simulink model "Sixteen_June_Sensors"  (R2022a)
settings: Solver=FixedStepAuto  StartTime=0.0  StopTime=80  RelTol=1e-3
settings Model: ExtModeTrigDuration=80  Creator=DevGunu  LastModifiedBy=DevGunu
settings OptimizationCC: EnhancedBackFolding=on  PassReuseOutputArgsAs=Individual arguments  ZeroExternalMemoryAtStartup=off  ZeroInternalMemoryAtStartup=off  MaxStackSize=64  OptimizeBlockOrder=speed  DifferentSizesBufferReuse=on  OptimizationCustomize=off  EfficientTunableParamExpr=on
settings DebuggingCC: ParameterTunabilityLossMsg=error
settings HardwareCC: ProdBitPerPointer=32  ProdBitPerSizeT=32  ProdBitPerPtrDiffT=32  ProdLargestAtomicInteger=Long  ProdWordSize=32  ProdHWDeviceType=ARM Compatible->ARM 9  UseEmbeddedCoderFeatures=off
settings SFSimCC: MATLABDynamicMemAlloc=off
settings RTWCC: SystemTargetFile=ert.tlc  HardwareBoard=PARROT Mambo  TemplateMakefile=ert_default_tmf  Toolchain=Sourcery G++ Lite GNU Toolchain for Drones
settings CodeAppCC: ForceParamTrailComments=on  IgnoreCustomStorageClasses=off  OperatorAnnotations=on  SimulinkDataObjDesc=on  SFDataObjDesc=on  InsertBlockDesc=on
settings ERTTargetCC: SupportNonInlinedSFcns=on

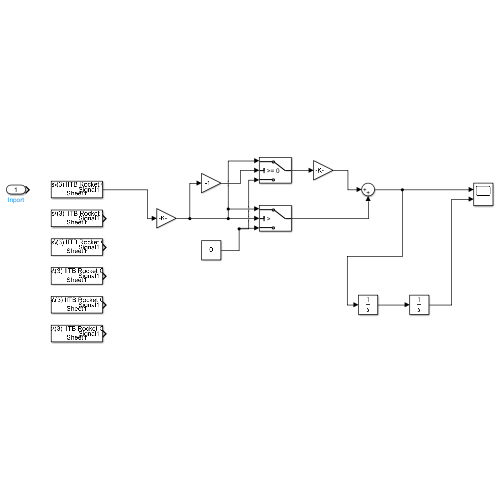
[thumbnail: Simulink's stored preview of the top-level diagram]
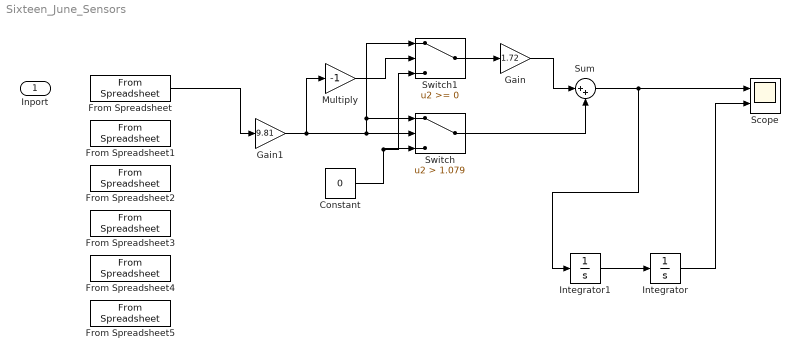
== system Sixteen_June_Sensors ==
  Inport : Inport
  Constant : Constant  Value=0
  From Spreadsheet : FromSpreadsheet  FileName=C:\Users\DevGunu\Desktop\Courses\(3) IITB Rocket Club\Flyte-Mini\Data Files\AccZ.xlsx  SampleTime=0.2
  From Spreadsheet1 : FromSpreadsheet  FileName=C:\Users\DevGunu\Desktop\Courses\(3) IITB Rocket Club\Flyte-Mini\Data Files\AccY.xlsx  SampleTime=0.2
  From Spreadsheet2 : FromSpreadsheet  FileName=C:\Users\DevGunu\Desktop\Courses\(3) IITB Rocket Club\Flyte-Mini\Data Files\AccX.xlsx  SampleTime=0.2
  From Spreadsheet3 : FromSpreadsheet  FileName=C:\Users\DevGunu\Desktop\Courses\(3) IITB Rocket Club\Flyte-Mini\Data Files\GyroZ.xlsx  SampleTime=0.2
  From Spreadsheet4 : FromSpreadsheet  FileName=C:\Users\DevGunu\Desktop\Courses\(3) IITB Rocket Club\Flyte-Mini\Data Files\GyroY.xlsx  SampleTime=0.2
  From Spreadsheet5 : FromSpreadsheet  FileName=C:\Users\DevGunu\Desktop\Courses\(3) IITB Rocket Club\Flyte-Mini\Data Files\GyroX.xlsx  SampleTime=0.2
  Gain : Gain  Gain=1.72
  Gain1 : Gain  Gain=9.81
  Integrator : Integrator
  Integrator1 : Integrator
  Multiply : Gain  Gain=-1
  Scope : Scope  NumInputPorts=2
  Sum : Sum  Inputs=|++
  Switch : Switch  Criteria=u2 > Threshold  Threshold=1.079  SaturateOnIntegerOverflow=off  InputSameDT=off
  Switch1 : Switch  SaturateOnIntegerOverflow=off  InputSameDT=off
  wires:
  Gain1/1 -> Multiply/1, Switch1/1, Switch/1, Switch/2
  Constant/1 -> Switch1/3, Switch/3
  Multiply/1 -> Switch1/2
  Switch1/1 -> Gain/1
  Switch/1 -> Sum/2
  Sum/1 -> Integrator1/1, Scope/1
  Integrator1/1 -> Integrator/1
  Integrator/1 -> Scope/2
  Gain/1 -> Sum/1
  From Spreadsheet/1 -> Gain1/1
